simulink model "EngineModel_scaled_10_6_2016_dynamics"  (R2013a)
settings: Solver=ode4  StartTime=0.0  StopTime=30  FixedStep=0.2  RelTol=1e-3
values from neighbouring files (symbols this model uses):
  Fanmap_2 = [1 1 1 1 1 1 1 1 1 1 275.724 325.4224 ... (330 elements, 10x3x11)]    [enginemaps2.mat]
  HPCompmap_2 = [1 1 1 1 1 1 1 1 1 1 32.390865 37.6623195 ... (330 elements, 10x3x11)]    [enginemaps2.mat]
  HPTurbinemap_2 = [0.24979968 0.24979968 0.24979968 0.24979968 0.24979968 0.24979968 0.24979968 0.24979968 0.24979968 0.24979968 0.004250667 0.005047667 ... (330 elements, 10x3x11)]    [enginemaps2.mat]
  LPCompmap_2 = [1 1 1 1 1 1 1 1 1 1 34.17260994 40.23277722 ... (330 elements, 10x3x11)]    [enginemaps2.mat]
  LPTurbinemap_2 = [0.665969797 0.665969797 0.665969797 0.665969797 0.665969797 0.665969797 0.665969797 0.665969797 0.00912 0.013173333 0.015706667 0.01672 ... (264 elements, 8x3x11)]    [enginemaps2.mat]
undefined symbols (not defined in the file or in its folder): acc_or_dec, acceleration, Adiabatic_compression_fan, Adiabatic_compression_HPC, Adiabatic_compression_LPC, coldnozzle, compression_ram, cond_f2, D, datatables, deceleration, hotnozzle, HPT1, if_Nth, if_Ntl, if_Z, LPT, performancedynOL, thermo_combustor, transient, turbo
libraries: dspmtrx3 x8, aerolibatmos2 x6, dspsigattribs x3, dspsolvers x2, dspfactors x1
(part 1 of 10)
settings Model: Creator=BES  LastModifiedBy=BES
settings SolverCC: ZeroCrossAlgorithm=Adaptive
settings DataIOCC: InitialState=load('enginemaps1.mat')  LimitDataPoints=off

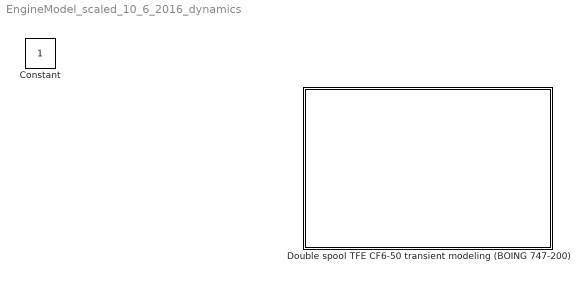
== system EngineModel_scaled_10_6_2016_dynamics ==
  Double spool TFE CF6-50 transient modeling (BOING 747-200) : Subsystem
      mask Display: image('b747.jpg')
  Constant : Constant  IOType=siggen

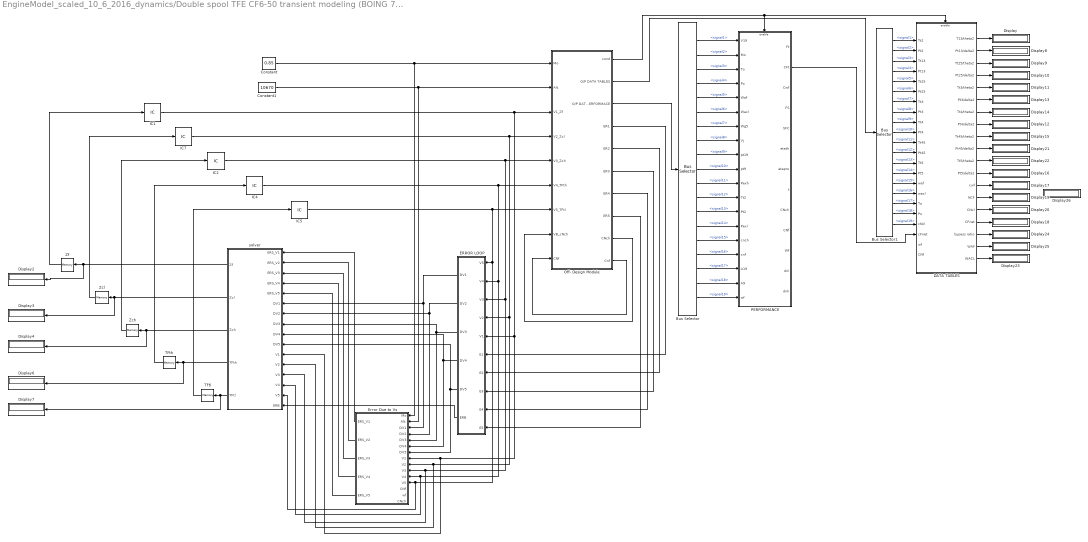
== system EngineModel_scaled_10_6_2016_dynamics/Double spool TFE CF6-50 transient modeling (BOING 747-200) ==
  Bus Selector : BusSelector  OutputSignals=signal1,signal2,signal3,signal4,signal5,signal6,signal7,signal8,signal9,signal10,signal11,signal12,signal13,signal14,signal15,signal16,signal17,signal18,signal19
  Bus Selector1 : BusSelector  OutputSignals=signal1,signal2,signal3,signal4,signal5,signal6,signal7,signal8,signal9,signal10,signal11,signal12,signal13,signal14,signal15,signal16,signal17,signal18,signal19
  Constant : Constant  Value=0.85
  Constant1 : Constant  Value=10670
  DATA TABLES : Subsystem
  Display{,2..4,6..26} (25 alike) : Display
  "ERROR LOOP " : Subsystem
  Error Due to Vs : Subsystem
  IC1 : InitialCondition  Value=0.838043
  IC2 : InitialCondition  Value=0.82992106
  IC4 : InitialCondition  Value=156.358278
  IC5 : InitialCondition  Value=677.9237033
  IC7 : InitialCondition  Value=0.8685268
  Off- Design Module : Subsystem
  PERFORMANCE : Subsystem
  TFth : Memory  X0=156
  TFtl : Memory  X0=674
  Zch : Memory  X0=0.83333
  Zcl : Memory  X0=0.83333
  Zf : Memory  X0=0.83333
  solver : Subsystem
  wires:
  Constant/1 -> Error Due to Vs/1(Mo), Off- Design Module/1(Mo)
  Constant1/1 -> Error Due to Vs/2(Alt.), Off- Design Module/2(Alt.)
  solver/1(Zf) -> Display2/1, Zf/1
  solver/2(Zcl) -> Display3/1, Zcl/1
  solver/3(Zch) -> Display4/1, Zch/1
  solver/4(TFth) -> TFth/1, Display6/1
  solver/5(TFtl) -> TFtl/1, Display7/1
  Off- Design Module/4(ER1) -> "ERROR LOOP "/6(E1)
  Off- Design Module/5(ER2) -> "ERROR LOOP "/7(E2)
  "ERROR LOOP "/6(ERB) -> solver/16(ERB)
  IC1/1 -> solver/11(V1), Error Due to Vs/8(V1), "ERROR LOOP "/5(V1), Off- Design Module/3(V1_Zf)
  IC7/1 -> solver/12(V2), Error Due to Vs/9(V2), "ERROR LOOP "/4(V2), Off- Design Module/4(V2_Zcl)
  IC2/1 -> solver/13(V3), Error Due to Vs/10(V3), "ERROR LOOP "/3(V3), Off- Design Module/5(V3_Zch)
  IC4/1 -> solver/14(V4), Error Due to Vs/11(V4), "ERROR LOOP "/2(V4), Off- Design Module/6(V4_TFth)
  IC5/1 -> solver/15(V5), Error Due to Vs/12(V5), "ERROR LOOP "/1(V5), Off- Design Module/7(V5_TFtl)
  Off- Design Module/1(cond) -> PERFORMANCE/Enable, DATA TABLES/Enable
  TFtl/1 -> IC5/1
  TFth/1 -> IC4/1
  Zch/1 -> IC2/1
  Zcl/1 -> IC7/1
  Zf/1 -> IC1/1
  Off- Design Module/2(O/P DATA TABLES) -> Bus Selector1/1
  Bus Selector1/1 -> DATA TABLES/1(Tt2)  "<signal1>"
  Bus Selector1/2 -> DATA TABLES/2(Pt2)  "<signal2>"
  Bus Selector1/3 -> DATA TABLES/3(Tt13)  "<signal3>"
  Bus Selector1/4 -> DATA TABLES/4(Pt13)  "<signal4>"
  Bus Selector1/5 -> DATA TABLES/5(Tt25)  "<signal5>"
  Bus Selector1/6 -> DATA TABLES/6(Pt25)  "<signal6>"
  Bus Selector1/7 -> DATA TABLES/7(Tt3)  "<signal7>"
  Bus Selector1/8 -> DATA TABLES/8(Pt3)  "<signal8>"
  Bus Selector1/9 -> DATA TABLES/9(Tt4)  "<signal9>"
  Bus Selector1/10 -> DATA TABLES/10(Pt4)  "<signal10>"
  Bus Selector1/11 -> DATA TABLES/11(Tt45)  "<signal11>"
  Bus Selector1/12 -> DATA TABLES/12(Pt45)  "<signal12>"
  Bus Selector1/13 -> DATA TABLES/13(Tt5)  "<signal13>"
  Bus Selector1/14 -> DATA TABLES/14(Pt5)  "<signal14>"
  Bus Selector1/15 -> DATA TABLES/15(waf)  "<signal15>"
  Bus Selector1/16 -> DATA TABLES/16(wacl)  "<signal16>"
  Bus Selector1/17 -> DATA TABLES/17(To)  "<signal17>"
  Bus Selector1/18 -> DATA TABLES/18(Po)  "<signal18>"
  Bus Selector1/19 -> DATA TABLES/19(cNcl)  "<signal19>"
  PERFORMANCE/2(CFt) -> DATA TABLES/20(cFnet)
  DATA TABLES/1(T13/theta2) -> Display/1
  DATA TABLES/2(Pt13/delta2) -> Display8/1
  DATA TABLES/3(Tt25/theta2) -> Display9/1
  DATA TABLES/4(Pt25/delta2) -> Display10/1
  DATA TABLES/5(Tt3/theta2) -> Display11/1
  DATA TABLES/6(Pt3/delta2) -> Display13/1
  DATA TABLES/7(Tt4/theta2) -> Display14/1
  DATA TABLES/8(Pt4/delta2) -> Display12/1
  DATA TABLES/9(Tt45/theta2) -> Display15/1
  DATA TABLES/10(Pt45/delta2) -> Display21/1
  DATA TABLES/11(Tt5/theta2) -> Display22/1
  DATA TABLES/12(Pt5/delta2) -> Display16/1
  DATA TABLES/13(cwf) -> Display17/1
  DATA TABLES/14(NCF) -> Display19/1
  DATA TABLES/15(CNcl) -> Display20/1
  DATA TABLES/16(CFnet) -> Display18/1
  DATA TABLES/17(bypass ratio) -> Display24/1
  DATA TABLES/18(WAF) -> Display25/1
  DATA TABLES/19(WACL) -> Display23/1
  Off- Design Module/6(ER3) -> "ERROR LOOP "/8(E3)
  Off- Design Module/7(ER4) -> "ERROR LOOP "/9(E4)
  Off- Design Module/8(ER5) -> "ERROR LOOP "/10(E5)
  "ERROR LOOP "/1(DV1) -> solver/6(DV1), Error Due to Vs/3(DV1)
  "ERROR LOOP "/2(DV2) -> solver/7(DV2), Error Due to Vs/4(DV2)
  "ERROR LOOP "/5(DV5) -> solver/10(DV5), Error Due to Vs/7(DV5)
  "ERROR LOOP "/4(DV4) -> solver/9(DV4), Error Due to Vs/6(DV4)
  "ERROR LOOP "/3(DV3) -> solver/8(DV3), Error Due to Vs/5(DV3)
  Error Due to Vs/1(ERS_V1) -> solver/1(ERS_V1)
  Error Due to Vs/2(ERS_V2) -> solver/2(ERS_V2)
  Error Due to Vs/3(ERS_V3) -> solver/3(ERS_V3)
  Error Due to Vs/4(ERS_V4) -> solver/4(ERS_V4)
  Error Due to Vs/5(ERS_V5) -> solver/5(ERS_V5)
  Bus Selector/1 -> PERFORMANCE/1(V19)  "<signal1>"
  Bus Selector/2 -> PERFORMANCE/2(Mo)  "<signal2>"
  Bus Selector/3 -> PERFORMANCE/3(To)  "<signal3>"
  Bus Selector/4 -> PERFORMANCE/4(Po)  "<signal4>"
  Bus Selector/5 -> PERFORMANCE/5(Waf)  "<signal5>"
  Bus Selector/6 -> PERFORMANCE/6(Wacl)  "<signal6>"
  Bus Selector/7 -> PERFORMANCE/7(Wg5)  "<signal7>"
  Bus Selector/8 -> PERFORMANCE/8(Vj)  "<signal8>"
  Bus Selector/9 -> PERFORMANCE/9(pt19)  "<signal9>"
  Bus Selector/10 -> PERFORMANCE/10(pt9)  "<signal10>"
  Bus Selector/11 -> PERFORMANCE/11(Pexh)  "<signal11>"
  Bus Selector/12 -> PERFORMANCE/12(Tt2)  "<signal12>"
  Bus Selector/13 -> PERFORMANCE/13(Pt2)  "<signal13>"
  Bus Selector/14 -> PERFORMANCE/14(Pexl)  "<signal14>"
  Bus Selector/15 -> PERFORMANCE/15(cnch)  "<signal15>"
  Bus Selector/16 -> PERFORMANCE/16(cnf)  "<signal16>"
  Bus Selector/17 -> PERFORMANCE/17(A19)  "<signal17>"
  Bus Selector/18 -> PERFORMANCE/18(A9)  "<signal18>"
  Bus Selector/19 -> PERFORMANCE/19(wf)  "<signal19>"
  Off- Design Module/3(O/P DATA FOR PERFORMACE) -> Bus Selector/1
  Off- Design Module/10(Cnf) -> Off- Design Module/9(CNf)
  Off- Design Module/9(CNch) -> Off- Design Module/8(VB_cNch)

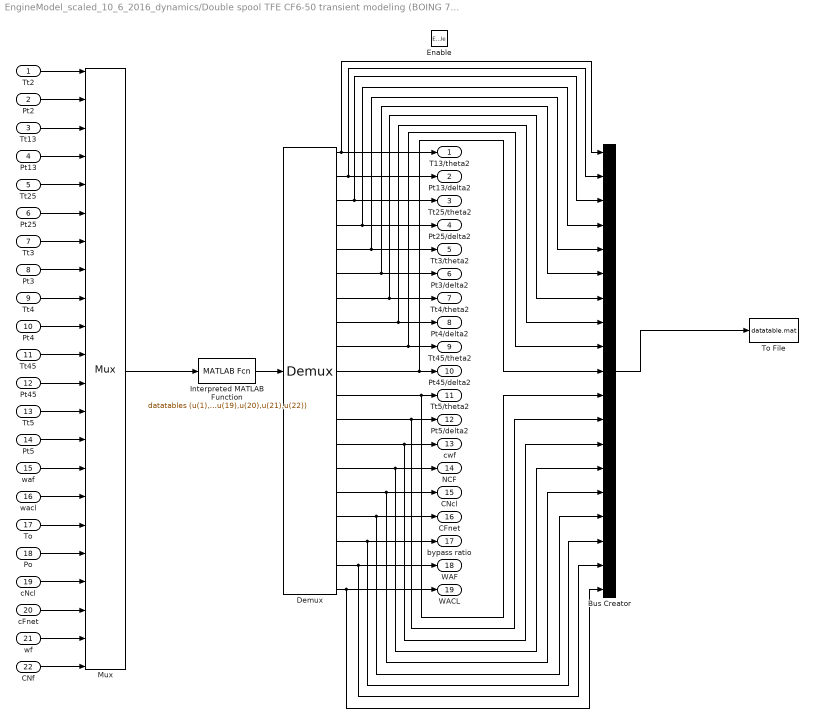
== system EngineModel_scaled_10_6_2016_dynamics/Double spool TFE CF6-50 transient modeling (BOING 747-200)/DATA TABLES ==
  Tt2 : Inport
  Pt2 : Inport  Port=2
  Tt13 : Inport  Port=3
  Pt13 : Inport  Port=4
  Tt25 : Inport  Port=5
  Pt25 : Inport  Port=6
  Tt3 : Inport  Port=7
  Pt3 : Inport  Port=8
  Tt4 : Inport  Port=9
  Pt4 : Inport  Port=10
  Tt45 : Inport  Port=11
  Pt45 : Inport  Port=12
  Tt5 : Inport  Port=13
  Pt5 : Inport  Port=14
  waf : Inport  Port=15
  wacl : Inport  Port=16
  To : Inport  Port=17
  Po : Inport  Port=18
  cNcl : Inport  Port=19
  cFnet : Inport  Port=20
  wf : Inport  Port=21
  CNf : Inport  Port=22
  Enable : EnablePort  StatesWhenEnabling=reset
  Bus Creator : BusCreator  Inputs=19
  Demux : Demux  Outputs=19
  Interpreted MATLAB Function : MATLABFcn  MATLABFcn=datatables (u(1),u(2),u(3),u(4),u(5),u(6),u(7),u(8),u(9),u(10),u(11),u(12),u(13),u(14),u(15),u(16),u(17),u(18),u(19),u(20),u(21),u(22))  OutputDimensions=19
  Mux : Mux  Inputs=22
      settings: DisplayOption=signals
  To File : ToFile  Filename=datatable.mat  MatrixName=bes
  T13/theta2 : Outport
  Pt13/delta2 : Outport  Port=2
  Tt25/theta2 : Outport  Port=3
  Pt25/delta2 : Outport  Port=4
  Tt3/theta2 : Outport  Port=5
  Pt3/delta2 : Outport  Port=6
  Tt4/theta2 : Outport  Port=7
  Pt4/delta2 : Outport  Port=8
  Tt45/theta2 : Outport  Port=9
  Pt45/delta2 : Outport  Port=10
  Tt5/theta2 : Outport  Port=11
  Pt5/delta2 : Outport  Port=12
  cwf : Outport  Port=13
  NCF : Outport  Port=14
  CNcl : Outport  Port=15
  CFnet : Outport  Port=16
  bypass ratio : Outport  Port=17
  WAF : Outport  Port=18
  WACL : Outport  Port=19
  wires:
  Pt5/1 -> Mux/14
  Tt5/1 -> Mux/13
  Pt45/1 -> Mux/12
  Tt45/1 -> Mux/11
  Pt4/1 -> Mux/10
  Pt3/1 -> Mux/8
  Tt3/1 -> Mux/7
  Pt25/1 -> Mux/6
  Tt25/1 -> Mux/5
  Pt13/1 -> Mux/4
  Tt13/1 -> Mux/3
  Pt2/1 -> Mux/2
  Tt2/1 -> Mux/1
  Interpreted MATLAB Function/1 -> Demux/1
  Mux/1 -> Interpreted MATLAB Function/1
  waf/1 -> Mux/15
  cNcl/1 -> Mux/19
  wacl/1 -> Mux/16
  To/1 -> Mux/17
  Po/1 -> Mux/18
  cFnet/1 -> Mux/20
  wf/1 -> Mux/21
  CNf/1 -> Mux/22
  Demux/1 -> Bus Creator/1, T13/theta2/1
  Demux/4 -> Bus Creator/4, Pt25/delta2/1
  Demux/5 -> Bus Creator/5, Tt3/theta2/1
  Demux/6 -> Bus Creator/6, Pt3/delta2/1
  Demux/7 -> Bus Creator/7, Tt4/theta2/1
  Demux/8 -> Bus Creator/8, Pt4/delta2/1
  Demux/9 -> Bus Creator/9, Tt45/theta2/1
  Demux/11 -> Bus Creator/11, Tt5/theta2/1
  Demux/12 -> Bus Creator/12, Pt5/delta2/1
  Demux/13 -> Bus Creator/13, cwf/1
  Demux/14 -> Bus Creator/14, NCF/1
  Demux/15 -> Bus Creator/15, CNcl/1
  Demux/16 -> Bus Creator/16, CFnet/1
  Demux/17 -> Bus Creator/17, bypass ratio/1
  Demux/18 -> Bus Creator/18, WAF/1
  Demux/19 -> Bus Creator/19, WACL/1
  Demux/2 -> Bus Creator/2, Pt13/delta2/1
  Bus Creator/1 -> To File/1
  Demux/3 -> Bus Creator/3, Tt25/theta2/1
  Demux/10 -> Bus Creator/10, Pt45/delta2/1
  Tt4/1 -> Mux/9

== system EngineModel_scaled_10_6_2016_dynamics/Double spool TFE CF6-50 transient modeling (BOING 747-200)/ERROR LOOP  ==
  V5 : Inport
  V4 : Inport  Port=2
  V3 : Inport  Port=3
  V2 : Inport  Port=4
  V1 : Inport  Port=5
  E1 : Inport  Port=6
  E2 : Inport  Port=7
  E3 : Inport  Port=8
  E4 : Inport  Port=9
  E5 : Inport  Port=10
  Constant : Constant  Value=0.005
  Constant1 : Constant  Value=100
  Display1 : Display
  Divide : Product  Inputs=*/
  Divide1 : Product  Inputs=*/
  Product{,1,3..5} (5 alike) : Product
  Vector Concatenate : Concatenate  NumInputs=5  Mode=Multidimensional array
  DV1 : Outport
  DV2 : Outport  Port=2
  DV3 : Outport  Port=3
  DV4 : Outport  Port=4
  DV5 : Outport  Port=5
  ERB : Outport  Port=6
  wires:
  Constant/1 -> Product5/1, Product4/1, Product3/1, Product1/1, Product/1
  V1/1 -> Product5/2
  V2/1 -> Product4/2
  V3/1 -> Product3/2
  Product3/1 -> DV3/1
  Product4/1 -> DV2/1
  Product5/1 -> DV1/1
  E1/1 -> Vector Concatenate/1
  E2/1 -> Vector Concatenate/2
  E3/1 -> Vector Concatenate/3
  E4/1 -> Vector Concatenate/4
  E5/1 -> Vector Concatenate/5
  Vector Concatenate/1 -> ERB/1, Display1/1
  Product/1 -> DV5/1
  Product1/1 -> DV4/1
  V5/1 -> Divide/1
  Constant1/1 -> Divide1/2, Divide/2
  Divide/1 -> Product/2
  V4/1 -> Divide1/1
  Divide1/1 -> Product1/2

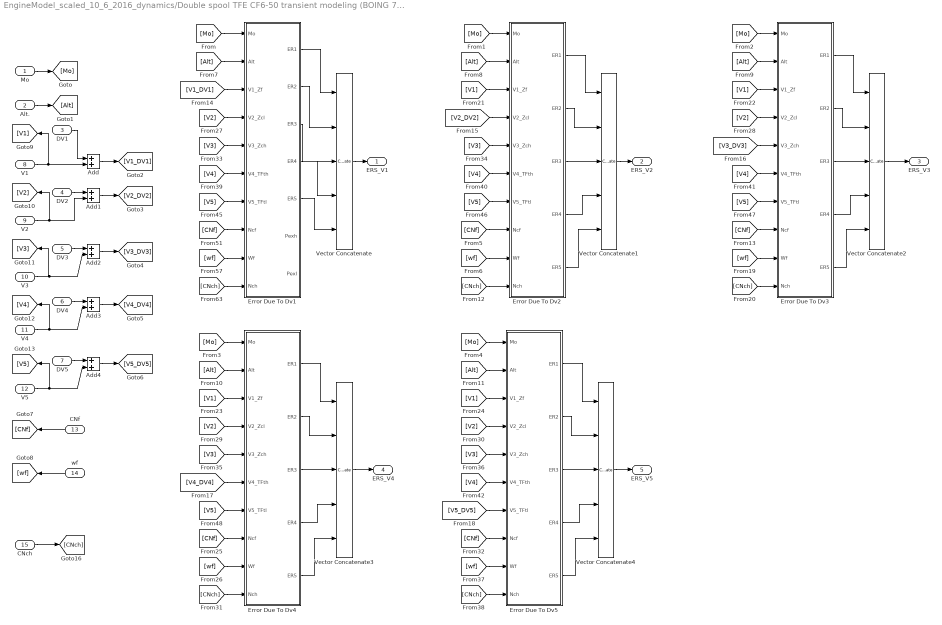
== system EngineModel_scaled_10_6_2016_dynamics/Double spool TFE CF6-50 transient modeling (BOING 747-200)/Error Due to Vs ==
  Mo : Inport
  Alt. : Inport  Port=2
  DV1 : Inport  Port=3
  DV2 : Inport  Port=4
  DV3 : Inport  Port=5
  DV4 : Inport  Port=6
  DV5 : Inport  Port=7
  V1 : Inport  Port=8
  V2 : Inport  Port=9
  V3 : Inport  Port=10
  V4 : Inport  Port=11
  V5 : Inport  Port=12
  CNf : Inport  Port=13
  wf : Inport  Port=14
  CNch : Inport  Port=15
  Add{,1..4} (5 alike) : Sum
  Error Due To Dv1 : Subsystem
  Error Due To Dv2 : Subsystem
  Error Due To Dv3 : Subsystem
  Error Due To Dv4 : Subsystem
  Error Due To Dv5 : Subsystem
  Vector Concatenate{,1..4} (5 alike) : Concatenate  NumInputs=5
  ERS_V1 : Outport
  ERS_V2 : Outport  Port=2
  ERS_V3 : Outport  Port=3
  ERS_V4 : Outport  Port=4
  ERS_V5 : Outport  Port=5
  wires:
  Vector Concatenate/1 -> ERS_V1/1
  Error Due To Dv1/1(ER1) -> Vector Concatenate/1
  Error Due To Dv1/2(ER2) -> Vector Concatenate/2
  Error Due To Dv1/4(ER4) -> Vector Concatenate/4
  Error Due To Dv1/5(ER5) -> Vector Concatenate/5
  DV1/1 -> Add/1
  V1/1 -> [V1], Add/2
  DV2/1 -> Add1/1
  DV3/1 -> Add2/1
  DV4/1 -> Add3/1
  DV5/1 -> Add4/1
  Mo/1 -> [Mo]
  [Mo] -> Error Due To Dv1/1(Mo)
  [Mo] -> Error Due To Dv2/1(Mo)
  [Mo] -> Error Due To Dv3/1(Mo)
  [Mo] -> Error Due To Dv4/1(Mo)
  [Mo] -> Error Due To Dv5/1(Mo)
  [Alt] -> Error Due To Dv1/2(Alt)
  Alt./1 -> [Alt]
  [Alt] -> Error Due To Dv2/2(Alt)
  [Alt] -> Error Due To Dv3/2(Alt)
  [Alt] -> Error Due To Dv4/2(Alt)
  [Alt] -> Error Due To Dv5/2(Alt)
  Add/1 -> [V1_DV1]
  Add1/1 -> [V2_DV2]
  Add2/1 -> [V3_DV3]
  Add3/1 -> [V4_DV4]
  Add4/1 -> [V5_DV5]
  [V2_DV2] -> Error Due To Dv2/4(V2_Zcl)
  [V3_DV3] -> Error Due To Dv3/5(V3_Zch)
  [V4_DV4] -> Error Due To Dv4/6(V4_TFth)
  [V5_DV5] -> Error Due To Dv5/7(V5_TFtl)
  V2/1 -> [V2], Add1/2
  V3/1 -> [V3], Add2/2
  V4/1 -> [V4], Add3/2
  V5/1 -> [V5], Add4/2
  CNch/1 -> [CNch]
  [V1] -> Error Due To Dv2/3(V1_Zf)
  [V1] -> Error Due To Dv3/3(V1_Zf)
  [V1] -> Error Due To Dv4/3(V1_Zf)
  [V1] -> Error Due To Dv5/3(V1_Zf)
  [V2] -> Error Due To Dv3/4(V2_Zcl)
  [V2] -> Error Due To Dv4/4(V2_Zcl)
  [V2] -> Error Due To Dv5/4(V2_Zcl)
  [V3] -> Error Due To Dv2/5(V3_Zch)
  [V3] -> Error Due To Dv4/5(V3_Zch)
  [V3] -> Error Due To Dv5/5(V3_Zch)
  [V4] -> Error Due To Dv2/6(V4_TFth)
  [V4] -> Error Due To Dv3/6(V4_TFth)
  [V4] -> Error Due To Dv5/6(V4_TFth)
  [V5] -> Error Due To Dv2/7(V5_TFtl)
  [V5] -> Error Due To Dv3/7(V5_TFtl)
  [V5] -> Error Due To Dv4/7(V5_TFtl)
  [CNf] -> Error Due To Dv2/8(Ncf)
  [CNf] -> Error Due To Dv3/8(Ncf)
  [CNf] -> Error Due To Dv4/8(Ncf)
  [CNf] -> Error Due To Dv5/8(Ncf)
  [wf] -> Error Due To Dv2/9(Wf)
  [wf] -> Error Due To Dv3/9(Wf)
  [wf] -> Error Due To Dv4/9(Wf)
  [wf] -> Error Due To Dv5/9(Wf)
  [CNch] -> Error Due To Dv2/10(Nch)
  [CNch] -> Error Due To Dv3/10(Nch)
  [CNch] -> Error Due To Dv4/10(Nch)
  [CNch] -> Error Due To Dv5/10(Nch)
  [V1_DV1] -> Error Due To Dv1/3(V1_Zf)
  [V2] -> Error Due To Dv1/4(V2_Zcl)
  [V3] -> Error Due To Dv1/5(V3_Zch)
  [V4] -> Error Due To Dv1/6(V4_TFth)
  [V5] -> Error Due To Dv1/7(V5_TFtl)
  [CNf] -> Error Due To Dv1/8(Ncf)
  [wf] -> Error Due To Dv1/9(Wf)
  [CNch] -> Error Due To Dv1/10(Nch)
  Error Due To Dv1/3(ER3) -> Vector Concatenate/3
  Vector Concatenate1/1 -> ERS_V2/1
  Error Due To Dv2/1(ER1) -> Vector Concatenate1/1
  Error Due To Dv2/2(ER2) -> Vector Concatenate1/2
  Error Due To Dv2/4(ER4) -> Vector Concatenate1/4
  Error Due To Dv2/5(ER5) -> Vector Concatenate1/5
  Error Due To Dv2/3(ER3) -> Vector Concatenate1/3
  Error Due To Dv3/1(ER1) -> Vector Concatenate2/1
  Error Due To Dv3/2(ER2) -> Vector Concatenate2/2
  Error Due To Dv3/4(ER4) -> Vector Concatenate2/4
  Error Due To Dv3/5(ER5) -> Vector Concatenate2/5
  Error Due To Dv3/3(ER3) -> Vector Concatenate2/3
  Vector Concatenate2/1 -> ERS_V3/1
  Error Due To Dv4/1(ER1) -> Vector Concatenate3/1
  Error Due To Dv4/2(ER2) -> Vector Concatenate3/2
  Error Due To Dv4/4(ER4) -> Vector Concatenate3/4
  Error Due To Dv4/5(ER5) -> Vector Concatenate3/5
  Error Due To Dv4/3(ER3) -> Vector Concatenate3/3
  Vector Concatenate3/1 -> ERS_V4/1
  Error Due To Dv5/1(ER1) -> Vector Concatenate4/1
  Error Due To Dv5/2(ER2) -> Vector Concatenate4/2
  Error Due To Dv5/4(ER4) -> Vector Concatenate4/4
  Error Due To Dv5/5(ER5) -> Vector Concatenate4/5
  Error Due To Dv5/3(ER3) -> Vector Concatenate4/3
  Vector Concatenate4/1 -> ERS_V5/1
  CNf/1 -> [CNf]
  wf/1 -> [wf]

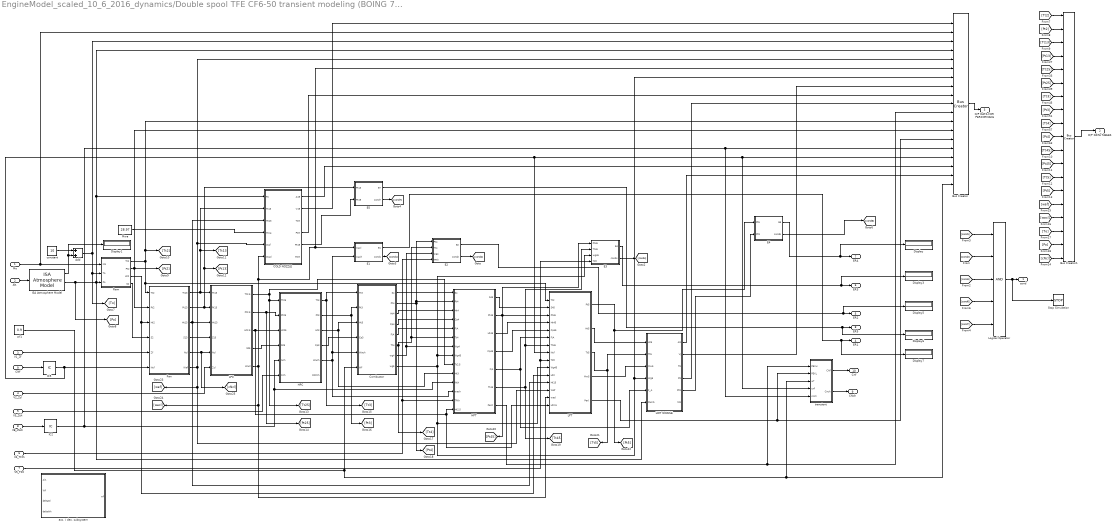
== system EngineModel_scaled_10_6_2016_dynamics/Double spool TFE CF6-50 transient modeling (BOING 747-200)/Off- Design Module ==
  Mo : Inport
  Alt. : Inport  Port=2
  V1_Zf : Inport  Port=3
  V2_Zcl : Inport  Port=4
  V3_Zch : Inport  Port=5
  V4_TFth : Inport  Port=6
  V5_TFtl : Inport  Port=7
  VB_cNch : Inport  Port=8
  CNf : Inport  Port=9
  Add : Sum
  Bus Creator : BusCreator  Inputs=19
  Bus Creator1 : BusCreator  Inputs=19
  COLD NOZZLE : Subsystem
  Combustor : Subsystem
  Display{,1,3,5..7} (6 alike) : Display
  E1 : Subsystem
  E2 : Subsystem
  E3 : Subsystem
  E4 : Subsystem
  E5 : Subsystem
  Fan : Subsystem
  HOT NOZZLE : Subsystem
  HPC : Subsystem
  HPT : Subsystem
  IC2 : InitialCondition
  IC5 : InitialCondition  Value=1.0141259
  ISA Atmosphere Model : aerolibatmos2/ISA Atmosphere Model  custom=on  g=9.8  gamma=1.4  R=287.0531  L=0.0065  h_trop=11000  h_strat=20000  rho0=1.225  P0=101325  T0=288.15  h0=0
  LPC : Subsystem
  LPT : Subsystem
  Logical Operator : Logic  Inputs=5  IconShape=distinctive  AllPortsSameDT=off  OutDataTypeStr=boolean
  Mwa : Constant  Value=28.97
  Ram : Subsystem
  Stop Simulation : Stop
  acc. / dec. subsystem : Subsystem
  constant : Constant  Value=10
  transient : Subsystem
  wf1 : Constant  Value=0.9
  cond : Outport
  O/P DATA TABLES : Outport  Port=2
  O/P DATA FOR PERFORMACE : Outport  Port=3
  ER1 : Outport  Port=4
  ER2 : Outport  Port=5
  ER3 : Outport  Port=6
  ER4 : Outport  Port=7
  ER5 : Outport  Port=8
  CNch : Outport  Port=9
  Cnf : Outport  Port=10
  wires:
  Alt./1 -> ISA Atmosphere Model/1
  Mo/1 -> Bus Creator/2, Ram/1(Mo)
  Add/1 -> Bus Creator/3, [To], Ram/2(To)
  ISA Atmosphere Model/3 -> [Po], HOT NOZZLE/6(Pamb), Ram/3(Po), Bus Creator/4, COLD NOZZLE/1(Po)
  constant/1 -> Add/1
  Ram/1(Tt2) -> [Tt2], Bus Creator/12, Fan/1(Tt2), LPT/1(Tt2)
  Ram/2(Pt2) -> [Pt2], Bus Creator/13, Fan/2(Pt2)
  HPC/2(Pt3) -> [Pt3], Combustor/2(Pt3)
  HPC/3(Ht3) -> HPT/10(Ht3), Combustor/3(Ht3)
  Combustor/2(Pt4) -> [Pt4], E2/1(Pt4), HPT/2(Pt4)
  Combustor/4(Cp4) -> HPT/4(Cp4)
  Combustor/5(F/A) -> HPT/5(F/A)
  Combustor/6(Tt4) -> [Tt4], E2/2(Tt4), HPT/6(Tt4)
  LPT/2(Ht5) -> HOT NOZZLE/1(Ht5)
  LPT/3(Tt5) -> [Tt5], HOT NOZZLE/2(Tt5)
  V1_Zf/1 -> Fan/5(Zf)
  V2_Zcl/1 -> LPC/6(Zcl)
  V3_Zch/1 -> HPC/6(Zch)
  VB_cNch/1 -> IC2/1
  V4_TFth/1 -> E2/4(TFth), HPT/13(TFth)
  Combustor/7(wg4) -> E2/3(wg4), HPT/7(Wg4)
  LPT/4(Mw5) -> HOT NOZZLE/3(Mw5)
  Fan/3(Ht13) -> LPC/3(Ht13), LPT/12(Ht13), COLD NOZZLE/3(Ht13)
  Mwa/1 -> COLD NOZZLE/4(Mwa)
  Fan/6(Waf) -> LPT/13(Waf), [waf], Bus Creator/5, COLD NOZZLE/5(Waf)
  LPC/5(Wacl) -> COLD NOZZLE/6(Wacl), Bus Creator/6, E1/1(wacl), LPT/14(wacl), [wacl]
  COLD NOZZLE/5(Pt19) -> E5/2(Pt19)
  LPC/3(Ht2.5) -> LPT/15(Ht2.5), HPT/14(Ht2.5), HPC/3(Ht25)
  LPT/1(Pt5) -> [Pt5], E4/1(Pt5)
  HOT NOZZLE/5(Pt9) -> E4/2(Pt9)
  Combustor/8(wg5) -> LPT/10(Wg45), Bus Creator/7, HOT NOZZLE/4(Wg5), E3/3(wg45), HPT/8(Wg45)
  Combustor/3(Ht4) -> HPT/3(Ht4)
  Combustor/1(S4) -> HPT/1(S4)
  Ram/4(S2) -> Fan/4(S2)
  Fan/5(Ncl) -> [cNcl], LPC/5(Ncl)
  Fan/4(S13) -> LPC/4(S13)
  LPC/4(S25) -> HPC/4(S25)
  HPC/5(Wach) -> HPT/12(wach), E1/2(wach), Combustor/5(Wach)
  HPT/1(S45) -> LPT/2(S45)
  HPT/2(Pt45) -> [Pt45], LPT/3(Pt45), E3/1(Pt45)
  HPT/3(Ht45) -> LPT/4(Ht45)
  HPT/4(Cp45) -> LPT/5(Cp45)
  HPT/6(Tt45) -> [Tt45], E3/2(Tt45), LPT/7(Tt45)
  V5_TFtl/1 -> E3/4(TFtl), LPT/9(TFtl)
  E4/1(E6) -> Display/1, ER4/1
  E3/1(E4) -> Display3/1, ER3/1
  E2/1(E2) -> Display5/1, ER2/1
  E5/1(E7) -> Display6/1, ER5/1
  E1/1(E1) -> Display7/1, ER1/1
  HOT NOZZLE/2(Vj) -> Bus Creator/8
  COLD NOZZLE/4(P19) -> Bus Creator/9
  HOT NOZZLE/4(P9) -> Bus Creator/10
  ISA Atmosphere Model/1 -> Display1/1, Add/2
  HOT NOZZLE/1(A9) -> Bus Creator/18
  COLD NOZZLE/2(V19) -> Bus Creator/1
  Bus Creator/1 -> O/P DATA FOR PERFORMACE/1
  E4/2(cond6) -> [cond6]
  E3/2(cond4) -> [cond4]
  E2/2(cond2) -> [cond2]
  E1/2(cond1) -> [cond1]
  E5/2("cond7 ") -> [cond7]
  Logical Operator/1 -> Stop Simulation/1, cond/1
  HPC/4(Cp3) -> Combustor/4(Cp3)
  [Tt2] -> Bus Creator1/1
  [Pt2] -> Bus Creator1/2
  [Tt13] -> Bus Creator1/3
  [Pt13] -> Bus Creator1/4
  [Tt25] -> Bus Creator1/5
  [Pt25] -> Bus Creator1/6
  [Tt3] -> Bus Creator1/7
  [Pt3] -> Bus Creator1/8
  [Tt4] -> Bus Creator1/9
  [Pt4] -> Bus Creator1/10
  [Tt45] -> Bus Creator1/11
  [Pt45] -> Bus Creator1/12
  [Tt5] -> Bus Creator1/13
  [Pt5] -> Bus Creator1/14
  [waf] -> Bus Creator1/15
  [wacl] -> Bus Creator1/16
  [To] -> Bus Creator1/17
  [Po] -> Bus Creator1/18
  Fan/1(Tt13) -> LPC/1(Tt13), [Tt13], COLD NOZZLE/2(Tt13)
  Fan/2(Pt13) -> [Pt13], E5/1(Pt13), LPC/2(Pt13)
  LPC/1(Tt2.5) -> HPT/9(Tt2.5), [Tt25], HPC/1(Tt25)
  LPC/2(Pt2.5) -> [Pt25], HPC/2(Pt25)
  HPC/1(Tt3) -> [Tt3], Combustor/1(Tt3)
  Bus Creator1/1 -> O/P DATA TABLES/1
  [cNcl] -> Bus Creator1/19
  HPT/5(F\A) -> HOT NOZZLE/5(F_A), LPT/6(F/A)
  [cond2] -> Logical Operator/2
  [cond1] -> Logical Operator/1
  [cond4] -> Logical Operator/3
  [cond6] -> Logical Operator/4
  [cond7] -> Logical Operator/5
  Ram/3(Ht2) -> Fan/3(Ht2), LPT/11(Ht2)
  CNf/1 -> IC5/1
  IC2/1 -> transient/5(cnch), Bus Creator/15, HPC/5(Nch), HPT/11(Nch)
  LPT/5(Pexl) -> transient/2(PEXL), Bus Creator/14
  wf1/1 -> transient/3(wf), Bus Creator/19, Combustor/6(Wf)
  COLD NOZZLE/1(A19) -> Bus Creator/17
  HPT/7(Pexh) -> transient/1(PEXH), Bus Creator/11
  IC5/1 -> LPT/8(Ncf), transient/4(cnf), Bus Creator/16, Fan/6(Ncf)
  transient/1(CNf) -> Cnf/1
  transient/2(Cnch) -> CNch/1

== system EngineModel_scaled_10_6_2016_dynamics/Double spool TFE CF6-50 transient modeling (BOING 747-200)/PERFORMANCE ==
  V19 : Inport
  Mo : Inport  Port=2
  To : Inport  Port=3
  Po : Inport  Port=4
  Waf : Inport  Port=5
  Wacl : Inport  Port=6
  Wg5 : Inport  Port=7
  Vj : Inport  Port=8
  pt19 : Inport  Port=9
  pt9 : Inport  Port=10
  Pexh : Inport  Port=11
  Tt2 : Inport  Port=12
  Pt2 : Inport  Port=13
  Pexl : Inport  Port=14
  cnch : Inport  Port=15
  cnf : Inport  Port=16
  A19 : Inport  Port=17
  A9 : Inport  Port=18
  wf : Inport  Port=19
  Enable : EnablePort  StatesWhenEnabling=reset
  Bus Creator : BusCreator  Inputs=6
  Demux : Demux  Outputs=13
  Interpreted MATLAB Function : MATLABFcn  MATLABFcn=performancedynOL(u(1),u(2),u(3),u(4),u(5),u(6),u(7),u(8),u(9),u(10),u(11),u(12),u(13),u(14),u(15),u(16),u(17),u(18),u(19),u(20),u(21),u(22))  OutputDimensions=13
  Mux : Mux  Inputs=22
      settings: DisplayOption=signals
  To File : ToFile  Filename=datatabledyn1.mat  MatrixName=bas1
  Ft : Outport
  CFt : Outport  Port=2
  Cwf : Outport  Port=3
  FS : Outport  Port=4
  SFC : Outport  Port=5
  etath : Outport  Port=6
  etapro : Outport  Port=7
  t : Outport  Port=8
  CNch : Outport  Port=9
  CNf : Outport  Port=10
  Wf : Outport  Port=11
  dnl : Outport  Port=12
  dnh : Outport  Port=13
  wires:
  Mux/1 -> Interpreted MATLAB Function/1
  Interpreted MATLAB Function/1 -> Demux/1
  V19/1 -> Mux/1
  Mo/1 -> Mux/2
  To/1 -> Mux/3
  Po/1 -> Mux/4
  Waf/1 -> Mux/5
  Wacl/1 -> Mux/6
  Wg5/1 -> Mux/7
  Vj/1 -> Mux/8
  pt19/1 -> Mux/9
  pt9/1 -> Mux/10
  Pexh/1 -> Mux/11
  Tt2/1 -> Mux/12
  Pt2/1 -> Mux/13
  Pexl/1 -> Mux/14
  cnch/1 -> Mux/15
  cnf/1 -> Mux/16
  A19/1 -> Mux/17
  A9/1 -> Mux/18
  wf/1 -> Mux/19
  Bus Creator/1 -> To File/1
  Demux/1 -> Ft/1
  Demux/2 -> CFt/1
  Demux/3 -> Cwf/1
  Demux/4 -> FS/1
  Demux/5 -> SFC/1
  Demux/6 -> etath/1
  Demux/7 -> etapro/1
  Demux/8 -> dnl/1
  Demux/9 -> dnh/1
  Demux/10 -> CNch/1
  Demux/11 -> CNf/1
  Demux/12 -> Wf/1
  Demux/13 -> t/1

== system EngineModel_scaled_10_6_2016_dynamics/Double spool TFE CF6-50 transient modeling (BOING 747-200)/solver ==
  ERS_V1 : Inport
  ERS_V2 : Inport  Port=2
  ERS_V3 : Inport  Port=3
  ERS_V4 : Inport  Port=4
  ERS_V5 : Inport  Port=5
  DV1 : Inport  Port=6
  DV2 : Inport  Port=7
  DV3 : Inport  Port=8
  DV4 : Inport  Port=9
  DV5 : Inport  Port=10
  V1 : Inport  Port=11
  V2 : Inport  Port=12
  V3 : Inport  Port=13
  V4 : Inport  Port=14
  V5 : Inport  Port=15
  ERB : Inport  Port=16
  " LU Inverse" : Subsystem  AncestorBlock=dspinverses/ LU Inverse  mask(LU Inverse){}
      mask help: Matrix inverse using LU factorization.
      mask Help: eval('blocksethelp');
      mask Display:
      | text(0.25,0.85,'General')
      | text(0.25,0.70,'Inverse')
      | text(0.35,0.25,'(LU)')
  Add{,1..4} (5 alike) : Sum
  Constant : Constant  Value=0.1
  Constant1 : Constant  Value=0
  Demux : Demux  Outputs=5
  Display{,1..2,4} (4 alike) : Display
  EMAT Concatenate : Concatenate  NumInputs=5  Mode=Multidimensional array  ConcatenateDimension=2
  EMAT New : Subsystem
  Matrix Multiply : Product  Multiplication=Matrix(*)
  Product : Product
  Subtract : Sum  Inputs=+-
  Zf : Outport
  Zcl : Outport  Port=2
  Zch : Outport  Port=3
  TFth : Outport  Port=4
  TFtl : Outport  Port=5
  wires:
  V1/1 -> Add/2
  V2/1 -> Add1/2
  V3/1 -> Add2/2
  V4/1 -> Add3/2
  V5/1 -> Add4/2
  " LU Inverse"/1(inv(A)) -> Matrix Multiply/1, Display1/1
  EMAT Concatenate/1 -> " LU Inverse"/1(A), Display/1
  Constant/1 -> Product/1
  Constant1/1 -> Subtract/1
  Matrix Multiply/1 -> Product/2, Display2/1
  Product/1 -> Demux/1, Display4/1
  Demux/1 -> Add/1
  Demux/2 -> Add1/1
  Demux/3 -> Add2/1
  Demux/4 -> Add3/1
  Demux/5 -> Add4/1
  ERS_V1/1 -> EMAT New/1(ERS_V1)
  ERS_V2/1 -> EMAT New/2(ERS_V2)
  ERS_V3/1 -> EMAT New/3(ERS_V3)
  ERS_V4/1 -> EMAT New/4(ERS_V4)
  ERS_V5/1 -> EMAT New/5(ERS_V5)
  ERB/1 -> EMAT New/6(ERB), Subtract/2
  DV1/1 -> EMAT New/7(DV1)
  DV2/1 -> EMAT New/8(DV2)
  DV3/1 -> EMAT New/9(DV3)
  DV4/1 -> EMAT New/10(DV4)
  DV5/1 -> EMAT New/11(DV5)
  EMAT New/1(EMAT1) -> EMAT Concatenate/1
  EMAT New/2(EMAT2) -> EMAT Concatenate/2
  EMAT New/3(EMAT3) -> EMAT Concatenate/3
  Subtract/1 -> Matrix Multiply/2
  Add/1 -> Zf/1
  Add1/1 -> Zcl/1
  Add2/1 -> Zch/1
  Add3/1 -> TFth/1
  Add4/1 -> TFtl/1
  EMAT New/4(EMAT4) -> EMAT Concatenate/4
  EMAT New/5(EMAT5) -> EMAT Concatenate/5

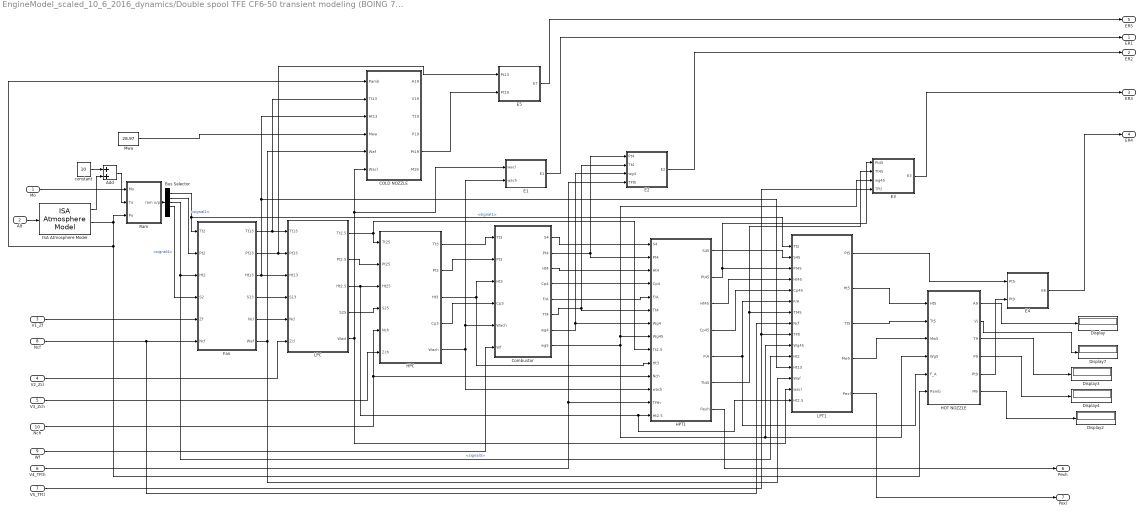
== system EngineModel_scaled_10_6_2016_dynamics/Double spool TFE CF6-50 transient modeling (BOING 747-200)/Error Due to Vs/Error Due To Dv1 ==
  Mo : Inport
  Alt : Inport  Port=2
  V1_Zf : Inport  Port=3
  V2_Zcl : Inport  Port=4
  V3_Zch : Inport  Port=5
  V4_TFth : Inport  Port=6
  V5_TFtl : Inport  Port=7
  Ncf : Inport  Port=8
  Wf : Inport  Port=9
  Nch : Inport  Port=10
  Add : Sum
  Bus Selector : BusSelector  OutputSignals=signal1,signal2,signal3,signal4,signal5
  COLD NOZZLE : Subsystem
  Combustor : Subsystem
  Display{,2..4,7} (5 alike) : Display
  E1 : Subsystem
  E2 : Subsystem
  E3 : Subsystem
  E4 : Subsystem
  E5 : Subsystem
  Fan : Subsystem
  HOT NOZZLE : Subsystem
  HPC : Subsystem
  HPT1 : Subsystem
  ISA Atmosphere Model : aerolibatmos2/ISA Atmosphere Model  custom=on  g=9.81  gamma=1.4  R=287  L=0.0065  h_trop=11000  h_strat=20000  rho0=1.225  P0=101325  T0=288  h0=0
  LPC : Subsystem
  LPT1 : Subsystem
  Mwa : Constant  Value=28.97
  Ram : Subsystem
  constant : Constant  Value=10
  ER1 : Outport
  ER2 : Outport  Port=2
  ER3 : Outport  Port=3
  ER4 : Outport  Port=4
  ER5 : Outport  Port=5
  Pexh : Outport  Port=6
  Pexl : Outport  Port=7
  wires:
  Alt/1 -> ISA Atmosphere Model/1
  Mo/1 -> Ram/1(Mo)
  ISA Atmosphere Model/1 -> Add/2
  Ram/1(ram o/p) -> Bus Selector/1
  ISA Atmosphere Model/3 -> Ram/3(Po), COLD NOZZLE/1(Pamb), HOT NOZZLE/6(Pamb)
  constant/1 -> Add/1
  Add/1 -> Ram/2(To)
  Bus Selector/1 -> LPT1/1(Tt2), Fan/1(Tt2)  "<signal1>"
  Bus Selector/2 -> Fan/2(Pt2)  "<signal2>"
  Fan/1(Tt13) -> LPC/1(Tt13), COLD NOZZLE/2(Tt13)
  Fan/2(Pt13) -> E5/1(Pt13), LPC/2(Pt13)
  LPC/1(Tt2.5) -> HPT1/9(Tt2.5), HPC/1(Tt25)
  LPC/2(Pt2.5) -> HPC/2(Pt25)
  HPC/1(Tt3) -> Combustor/1(Tt3)
  HPC/2(Pt3) -> Combustor/2(Pt3)
  HPC/3(Ht3) -> HPT1/10(Ht3), Combustor/3(Ht3)
  Combustor/2(Pt4) -> E2/1(Pt4), HPT1/2(Pt4)
  Combustor/4(Cp4) -> HPT1/4(Cp4)
  Combustor/5(F/A) -> HPT1/5(F/A)
  Combustor/6(Tt4) -> HPT1/6(Tt4), E2/2(Tt4)
  LPT1/2(Ht5) -> HOT NOZZLE/1(Ht5)
  LPT1/3(Tt5) -> HOT NOZZLE/2(Tt5)
  V1_Zf/1 -> Fan/5(Zf)
  Ncf/1 -> LPT1/8(Ncf), Fan/6(Ncf)
  V2_Zcl/1 -> LPC/6(Zcl)
  V3_Zch/1 -> HPC/6(Zch)
  Nch/1 -> HPC/5(Nch), HPT1/11(Nch)
  Wf/1 -> Combustor/6(Wf)
  V4_TFth/1 -> E2/4(TFth), HPT1/13(TFth)
  Combustor/7(wg4) -> E2/3(wg4), HPT1/7(Wg4)
  LPT1/4(Mw5) -> HOT NOZZLE/3(Mw5)
  Fan/3(Ht13) -> COLD NOZZLE/3(Ht13), LPT1/12(Ht13), LPC/3(Ht13)
  Mwa/1 -> COLD NOZZLE/4(Mwa)
  Fan/6(Waf) -> LPT1/13(Waf), COLD NOZZLE/5(Waf)
  LPC/5(Wacl) -> E1/1(wacl), COLD NOZZLE/6(Wacl), LPT1/14(wacl)
  COLD NOZZLE/5(Pt19) -> E5/2(Pt19)
  LPC/3(Ht2.5) -> HPC/3(Ht25), LPT1/15(Ht2.5), HPT1/14(Ht2.5)
  LPT1/1(Pt5) -> E4/1(Pt5)
  HOT NOZZLE/5(Pt9) -> E4/2(Pt9)
  Combustor/8(wg5) -> E3/3(wg45), HPT1/8(Wg45), LPT1/10(Wg45), HOT NOZZLE/4(Wg5)
  Combustor/3(Ht4) -> HPT1/3(Ht4)
  Combustor/1(S4) -> HPT1/1(S4)
  HOT NOZZLE/1(A9) -> Display/1
  HOT NOZZLE/2(Vj) -> Display7/1
  HOT NOZZLE/3(T9) -> Display3/1
  HOT NOZZLE/4(P9) -> Display4/1
  HOT NOZZLE/6(M9) -> Display2/1
  Bus Selector/3 -> Fan/3(Ht2), LPT1/11(Ht2)  "<signal3>"
  Bus Selector/4 -> Fan/4(S2)  "<signal4>"
  Fan/5(Ncl) -> LPC/5(Ncl)
  Fan/4(S13) -> LPC/4(S13)
  LPC/4(S25) -> HPC/4(S25)
  HPC/5(Wach) -> HPT1/12(wach), Combustor/5(Wach), E1/2(wach)
  HPT1/1(S45) -> LPT1/2(S45)
  HPT1/2(Pt45) -> LPT1/3(Pt45), E3/1(Pt45)
  HPT1/3(Ht45) -> LPT1/4(Ht45)
  HPT1/4(Cp45) -> LPT1/5(Cp45)
  HPT1/6(Tt45) -> LPT1/7(Tt45), E3/2(Tt45)
  HPT1/5(F\A) -> LPT1/6(F/A), HOT NOZZLE/5(F_A)
  V5_TFtl/1 -> LPT1/9(TFtl), E3/4(TFtl)
  E4/1(E6) -> ER4/1
  E3/1(E3) -> ER3/1
  E2/1(E2) -> ER2/1
  E1/1(E1) -> ER1/1
  E5/1(E7) -> ER5/1
  HPC/4(Cp3) -> Combustor/4(Cp3)
  HPT1/7(Pexh) -> Pexh/1
  LPT1/5(Pexl) -> Pexl/1

== system EngineModel_scaled_10_6_2016_dynamics/Double spool TFE CF6-50 transient modeling (BOING 747-200)/Error Due to Vs/Error Due To Dv2 ==
  Mo : Inport
  Alt : Inport  Port=2
  V1_Zf : Inport  Port=3
  V2_Zcl : Inport  Port=4
  V3_Zch : Inport  Port=5
  V4_TFth : Inport  Port=6
  V5_TFtl : Inport  Port=7
  Ncf : Inport  Port=8
  Wf : Inport  Port=9
  Nch : Inport  Port=10
  Add : Sum
  Bus Selector : BusSelector  OutputSignals=signal1,signal2,signal3,signal4,signal5
  COLD NOZZLE : Subsystem
  Combustor : Subsystem
  Display{,2..4,7} (5 alike) : Display
  E1 : Subsystem
  E2 : Subsystem
  E3 : Subsystem
  E4 : Subsystem
  E5 : Subsystem
  Fan : Subsystem
  HOT NOZZLE : Subsystem
  HPC : Subsystem
  HPT : Subsystem
  ISA Atmosphere Model : aerolibatmos2/ISA Atmosphere Model  custom=on  g=9.81  gamma=1.4  R=287  L=0.0065  h_trop=11000  h_strat=20000  rho0=1.225  P0=101325  T0=288  h0=0
  LPC : Subsystem
  LPT : Subsystem
  Mwa : Constant  Value=28.97
  Ram : Subsystem
  constant : Constant  Value=10
  ER1 : Outport
  ER2 : Outport  Port=2
  ER3 : Outport  Port=3
  ER4 : Outport  Port=4
  ER5 : Outport  Port=5
  wires:
  HPC/4(Cp3) -> Combustor/4(Cp3)
  E5/1(E7) -> ER5/1
  E1/1(E1) -> ER1/1
  E2/1(E2) -> ER2/1
  E3/1(E3) -> ER3/1
  E4/1(E6) -> ER4/1
  V5_TFtl/1 -> E3/4(TFtl), LPT/9(TFtl)
  HPT/6(F\A) -> HOT NOZZLE/5(F_A), LPT/6(F/A)
  HPT/7(Tt45) -> E3/2(Tt45), LPT/7(Tt45)
  HPT/5(Cp45) -> LPT/5(Cp45)
  HPT/4(Ht45) -> LPT/4(Ht45)
  HPT/3(Pt45) -> LPT/3(Pt45), E3/1(Pt45)
  HPT/2(S45) -> LPT/2(S45)
  HPC/5(Wach) -> HPT/12(wach), E1/2(wach), Combustor/5(Wach)
  LPC/4(S25) -> HPC/4(S25)
  Fan/4(S13) -> LPC/4(S13)
  Fan/5(Ncl) -> LPC/5(Ncl)
  Bus Selector/4 -> Fan/4(S2)  "<signal4>"
  Bus Selector/3 -> Fan/3(Ht2)  "<signal3>"
  HOT NOZZLE/6(M9) -> Display2/1
  HOT NOZZLE/4(P9) -> Display4/1
  HOT NOZZLE/3(T9) -> Display3/1
  HOT NOZZLE/2(Vj) -> Display7/1
  HOT NOZZLE/1(A9) -> Display/1
  Combustor/1(S4) -> HPT/1(S4)
  Combustor/3(Ht4) -> HPT/3(Ht4)
  Combustor/8(wg5) -> HOT NOZZLE/4(Wg5), HPT/8(Wg45), E3/3(wg45)
  HOT NOZZLE/5(Pt9) -> E4/2(Pt9)
  LPT/2(Pt5) -> E4/1(Pt5)
  LPC/3(Ht2.5) -> HPC/3(Ht25)
  COLD NOZZLE/5(Pt19) -> E5/2(Pt19)
  LPC/5(Wacl) -> E1/1(wacl), COLD NOZZLE/6(Wacl)
  Fan/6(Waf) -> COLD NOZZLE/5(Waf)
  Mwa/1 -> COLD NOZZLE/4(Mwa)
  Fan/3(Ht13) -> LPC/3(Ht13), COLD NOZZLE/3(Ht13)
  LPT/5(Mw5) -> HOT NOZZLE/3(Mw5)
  Combustor/7(wg4) -> HPT/7(Wg4), E2/3(wg4)
  V4_TFth/1 -> HPT/13(TFth), E2/4(TFth)
  Wf/1 -> Combustor/6(Wf)
  Nch/1 -> HPC/5(Nch), HPT/10(Nch)
  V3_Zch/1 -> HPC/6(Zch)
  V2_Zcl/1 -> LPC/6(Zcl)
  Ncf/1 -> Fan/6(Ncf), LPT/8(Ncf)
  V1_Zf/1 -> Fan/5(Zf)
  LPT/4(Tt5) -> HOT NOZZLE/2(Tt5)
  LPT/3(Ht5) -> HOT NOZZLE/1(Ht5)
  Combustor/6(Tt4) -> HPT/6(Tt4), E2/2(Tt4)
  Combustor/5(F/A) -> HPT/5(F/A)
  Combustor/4(Cp4) -> HPT/4(Cp4)
  Combustor/2(Pt4) -> HPT/2(Pt4), E2/1(Pt4)
  HPC/3(Ht3) -> HPT/11(Ht3), Combustor/3(Ht3)
  HPC/2(Pt3) -> Combustor/2(Pt3)
  HPC/1(Tt3) -> Combustor/1(Tt3)
  LPC/2(Pt2.5) -> HPC/2(Pt25)
  LPC/1(Tt2.5) -> HPT/9(Tt2.5), HPC/1(Tt25)
  Fan/2(Pt13) -> LPC/2(Pt13), E5/1(Pt13)
  Fan/1(Tt13) -> COLD NOZZLE/2(Tt13), LPC/1(Tt13)
  Bus Selector/2 -> Fan/2(Pt2)  "<signal2>"
  Bus Selector/1 -> LPT/1(Tt2), Fan/1(Tt2)  "<signal1>"
  Add/1 -> Ram/2(To)
  constant/1 -> Add/1
  ISA Atmosphere Model/3 -> HOT NOZZLE/6(Pamb), COLD NOZZLE/1(Pamb), Ram/3(Po)
  Ram/1(ram o/p) -> Bus Selector/1
  ISA Atmosphere Model/1 -> Add/2
  Mo/1 -> Ram/1(Mo)
  Alt/1 -> ISA Atmosphere Model/1

== system EngineModel_scaled_10_6_2016_dynamics/Double spool TFE CF6-50 transient modeling (BOING 747-200)/Error Due to Vs/Error Due To Dv3 ==
  Mo : Inport
  Alt : Inport  Port=2
  V1_Zf : Inport  Port=3
  V2_Zcl : Inport  Port=4
  V3_Zch : Inport  Port=5
  V4_TFth : Inport  Port=6
  V5_TFtl : Inport  Port=7
  Ncf : Inport  Port=8
  Wf : Inport  Port=9
  Nch : Inport  Port=10
  Add : Sum
  Bus Selector : BusSelector  OutputSignals=signal1,signal2,signal3,signal4,signal5
  COLD NOZZLE : Subsystem
  Combustor : Subsystem
  Display{,2..4,7} (5 alike) : Display
  E1 : Subsystem
  E2 : Subsystem
  E3 : Subsystem
  E4 : Subsystem
  E5 : Subsystem
  Fan : Subsystem
  HOT NOZZLE : Subsystem
  HPC : Subsystem
  HPT : Subsystem
  ISA Atmosphere Model : aerolibatmos2/ISA Atmosphere Model  custom=on  g=9.81  gamma=1.4  R=287  L=0.0065  h_trop=11000  h_strat=20000  rho0=1.225  P0=101325  T0=288  h0=0
  LPC : Subsystem
  LPT : Subsystem
  Mwa : Constant  Value=28.97
  Ram : Subsystem
  constant : Constant  Value=10
  ER1 : Outport
  ER2 : Outport  Port=2
  ER3 : Outport  Port=3
  ER4 : Outport  Port=4
  ER5 : Outport  Port=5
  wires:
  Alt/1 -> ISA Atmosphere Model/1
  Mo/1 -> Ram/1(Mo)
  ISA Atmosphere Model/1 -> Add/2
  Ram/1(ram o/p) -> Bus Selector/1
  ISA Atmosphere Model/3 -> Ram/3(Po), COLD NOZZLE/1(Pamb), HOT NOZZLE/6(Pamb)
  constant/1 -> Add/1
  Add/1 -> Ram/2(To)
  Bus Selector/1 -> Fan/1(Tt2), LPT/1(Tt2)  "<signal1>"
  Bus Selector/2 -> Fan/2(Pt2)  "<signal2>"
  Fan/1(Tt13) -> LPC/1(Tt13), COLD NOZZLE/2(Tt13)
  Fan/2(Pt13) -> E5/1(Pt13), LPC/2(Pt13)
  LPC/1(Tt2.5) -> HPC/1(Tt25), HPT/9(Tt2.5)
  LPC/2(Pt2.5) -> HPC/2(Pt25)
  HPC/1(Tt3) -> Combustor/1(Tt3)
  HPC/2(Pt3) -> Combustor/2(Pt3)
  HPC/3(Ht3) -> Combustor/3(Ht3), HPT/11(Ht3)
  Combustor/2(Pt4) -> E2/1(Pt4), HPT/2(Pt4)
  Combustor/4(Cp4) -> HPT/4(Cp4)
  Combustor/5(F/A) -> HPT/5(F/A)
  Combustor/6(Tt4) -> E2/2(Tt4), HPT/6(Tt4)
  LPT/3(Ht5) -> HOT NOZZLE/1(Ht5)
  LPT/4(Tt5) -> HOT NOZZLE/2(Tt5)
  V1_Zf/1 -> Fan/5(Zf)
  Ncf/1 -> LPT/8(Ncf), Fan/6(Ncf)
  V2_Zcl/1 -> LPC/6(Zcl)
  V3_Zch/1 -> HPC/6(Zch)
  Nch/1 -> HPT/10(Nch), HPC/5(Nch)
  Wf/1 -> Combustor/6(Wf)
  V4_TFth/1 -> E2/4(TFth), HPT/13(TFth)
  Combustor/7(wg4) -> E2/3(wg4), HPT/7(Wg4)
  LPT/5(Mw5) -> HOT NOZZLE/3(Mw5)
  Fan/3(Ht13) -> COLD NOZZLE/3(Ht13), LPC/3(Ht13)
  Mwa/1 -> COLD NOZZLE/4(Mwa)
  Fan/6(Waf) -> COLD NOZZLE/5(Waf)
  LPC/5(Wacl) -> COLD NOZZLE/6(Wacl), E1/1(wacl)
  COLD NOZZLE/5(Pt19) -> E5/2(Pt19)
  LPC/3(Ht2.5) -> HPC/3(Ht25)
  LPT/2(Pt5) -> E4/1(Pt5)
  HOT NOZZLE/5(Pt9) -> E4/2(Pt9)
  Combustor/8(wg5) -> E3/3(wg45), HPT/8(Wg45), HOT NOZZLE/4(Wg5)
  Combustor/3(Ht4) -> HPT/3(Ht4)
  Combustor/1(S4) -> HPT/1(S4)
  HOT NOZZLE/1(A9) -> Display/1
  HOT NOZZLE/2(Vj) -> Display7/1
  HOT NOZZLE/3(T9) -> Display3/1
  HOT NOZZLE/4(P9) -> Display4/1
  HOT NOZZLE/6(M9) -> Display2/1
  Bus Selector/3 -> Fan/3(Ht2)  "<signal3>"
  Bus Selector/4 -> Fan/4(S2)  "<signal4>"
  Fan/5(Ncl) -> LPC/5(Ncl)
  Fan/4(S13) -> LPC/4(S13)
  LPC/4(S25) -> HPC/4(S25)
  HPC/5(Wach) -> Combustor/5(Wach), E1/2(wach), HPT/12(wach)
  HPT/2(S45) -> LPT/2(S45)
  HPT/3(Pt45) -> E3/1(Pt45), LPT/3(Pt45)
  HPT/4(Ht45) -> LPT/4(Ht45)
  HPT/5(Cp45) -> LPT/5(Cp45)
  HPT/7(Tt45) -> LPT/7(Tt45), E3/2(Tt45)
  HPT/6(F\A) -> LPT/6(F/A), HOT NOZZLE/5(F_A)
  V5_TFtl/1 -> LPT/9(TFtl), E3/4(TFtl)
  E4/1(E6) -> ER4/1
  E3/1(E3) -> ER3/1
  E2/1(E2) -> ER2/1
  E1/1(E1) -> ER1/1
  E5/1(E7) -> ER5/1
  HPC/4(Cp3) -> Combustor/4(Cp3)

== system EngineModel_scaled_10_6_2016_dynamics/Double spool TFE CF6-50 transient modeling (BOING 747-200)/Error Due to Vs/Error Due To Dv4 ==
  Mo : Inport
  Alt : Inport  Port=2
  V1_Zf : Inport  Port=3
  V2_Zcl : Inport  Port=4
  V3_Zch : Inport  Port=5
  V4_TFth : Inport  Port=6
  V5_TFtl : Inport  Port=7
  Ncf : Inport  Port=8
  Wf : Inport  Port=9
  Nch : Inport  Port=10
  Add : Sum
  Bus Selector : BusSelector  OutputSignals=signal1,signal2,signal3,signal4,signal5
  COLD NOZZLE : Subsystem
  Combustor : Subsystem
  Display{,2..4,7} (5 alike) : Display
  E1 : Subsystem
  E2 : Subsystem
  E3 : Subsystem
  E4 : Subsystem
  E5 : Subsystem
  Fan : Subsystem
  HOT NOZZLE : Subsystem
  HPC : Subsystem
  HPT : Subsystem
  ISA Atmosphere Model : aerolibatmos2/ISA Atmosphere Model  custom=on  g=9.81  gamma=1.4  R=287  L=0.0065  h_trop=11000  h_strat=20000  rho0=1.225  P0=101325  T0=288  h0=0
  LPC : Subsystem
  LPT : Subsystem
  Mwa : Constant  Value=28.97
  Ram : Subsystem
  constant : Constant  Value=10
  ER1 : Outport
  ER2 : Outport  Port=2
  ER3 : Outport  Port=3
  ER4 : Outport  Port=4
  ER5 : Outport  Port=5
  wires:
  HPC/4(Cp3) -> Combustor/4(Cp3)
  E5/1(E7) -> ER5/1
  E1/1(E1) -> ER1/1
  E2/1(E2) -> ER2/1
  E3/1(E3) -> ER3/1
  E4/1(E6) -> ER4/1
  V5_TFtl/1 -> E3/4(TFtl), LPT/9(TFtl)
  HPT/6(F\A) -> HOT NOZZLE/5(F_A), LPT/6(F/A)
  HPT/7(Tt45) -> E3/2(Tt45), LPT/7(Tt45)
  HPT/5(Cp45) -> LPT/5(Cp45)
  HPT/4(Ht45) -> LPT/4(Ht45)
  HPT/3(Pt45) -> LPT/3(Pt45), E3/1(Pt45)
  HPT/2(S45) -> LPT/2(S45)
  HPC/5(Wach) -> HPT/12(wach), E1/2(wach), Combustor/5(Wach)
  LPC/4(S25) -> HPC/4(S25)
  Fan/4(S13) -> LPC/4(S13)
  Fan/5(Ncl) -> LPC/5(Ncl)
  Bus Selector/4 -> Fan/4(S2)  "<signal4>"
  Bus Selector/3 -> Fan/3(Ht2)  "<signal3>"
  HOT NOZZLE/6(M9) -> Display2/1
  HOT NOZZLE/4(P9) -> Display4/1
  HOT NOZZLE/3(T9) -> Display3/1
  HOT NOZZLE/2(Vj) -> Display7/1
  HOT NOZZLE/1(A9) -> Display/1
  Combustor/1(S4) -> HPT/1(S4)
  Combustor/3(Ht4) -> HPT/3(Ht4)
  Combustor/8(wg5) -> HOT NOZZLE/4(Wg5), HPT/8(Wg45), E3/3(wg45)
  HOT NOZZLE/5(Pt9) -> E4/2(Pt9)
  LPT/2(Pt5) -> E4/1(Pt5)
  LPC/3(Ht2.5) -> HPC/3(Ht25)
  COLD NOZZLE/5(Pt19) -> E5/2(Pt19)
  LPC/5(Wacl) -> E1/1(wacl), COLD NOZZLE/6(Wacl)
  Fan/6(Waf) -> COLD NOZZLE/5(Waf)
  Mwa/1 -> COLD NOZZLE/4(Mwa)
  Fan/3(Ht13) -> LPC/3(Ht13), COLD NOZZLE/3(Ht13)
  LPT/5(Mw5) -> HOT NOZZLE/3(Mw5)
  Combustor/7(wg4) -> HPT/7(Wg4), E2/3(wg4)
  V4_TFth/1 -> HPT/13(TFth), E2/4(TFth)
  Wf/1 -> Combustor/6(Wf)
  Nch/1 -> HPC/5(Nch), HPT/10(Nch)
  V3_Zch/1 -> HPC/6(Zch)
  V2_Zcl/1 -> LPC/6(Zcl)
  Ncf/1 -> Fan/6(Ncf), LPT/8(Ncf)
  V1_Zf/1 -> Fan/5(Zf)
  LPT/4(Tt5) -> HOT NOZZLE/2(Tt5)
  LPT/3(Ht5) -> HOT NOZZLE/1(Ht5)
  Combustor/6(Tt4) -> HPT/6(Tt4), E2/2(Tt4)
  Combustor/5(F/A) -> HPT/5(F/A)
  Combustor/4(Cp4) -> HPT/4(Cp4)
  Combustor/2(Pt4) -> HPT/2(Pt4), E2/1(Pt4)
  HPC/3(Ht3) -> HPT/11(Ht3), Combustor/3(Ht3)
  HPC/2(Pt3) -> Combustor/2(Pt3)
  HPC/1(Tt3) -> Combustor/1(Tt3)
  LPC/2(Pt2.5) -> HPC/2(Pt25)
  LPC/1(Tt2.5) -> HPT/9(Tt2.5), HPC/1(Tt25)
  Fan/2(Pt13) -> LPC/2(Pt13), E5/1(Pt13)
  Fan/1(Tt13) -> COLD NOZZLE/2(Tt13), LPC/1(Tt13)
  Bus Selector/2 -> Fan/2(Pt2)  "<signal2>"
  Bus Selector/1 -> LPT/1(Tt2), Fan/1(Tt2)  "<signal1>"
  Add/1 -> Ram/2(To)
  constant/1 -> Add/1
  ISA Atmosphere Model/3 -> HOT NOZZLE/6(Pamb), COLD NOZZLE/1(Pamb), Ram/3(Po)
  Ram/1(ram o/p) -> Bus Selector/1
  ISA Atmosphere Model/1 -> Add/2
  Mo/1 -> Ram/1(Mo)
  Alt/1 -> ISA Atmosphere Model/1

== system EngineModel_scaled_10_6_2016_dynamics/Double spool TFE CF6-50 transient modeling (BOING 747-200)/Error Due to Vs/Error Due To Dv5 ==
  Mo : Inport
  Alt : Inport  Port=2
  V1_Zf : Inport  Port=3
  V2_Zcl : Inport  Port=4
  V3_Zch : Inport  Port=5
  V4_TFth : Inport  Port=6
  V5_TFtl : Inport  Port=7
  Ncf : Inport  Port=8
  Wf : Inport  Port=9
  Nch : Inport  Port=10
  Add : Sum
  Bus Selector : BusSelector  OutputSignals=signal1,signal2,signal3,signal4,signal5
  COLD NOZZLE : Subsystem
  Combustor : Subsystem
  Display{,2..4,7} (5 alike) : Display
  E1 : Subsystem
  E2 : Subsystem
  E3 : Subsystem
  E4 : Subsystem
  E5 : Subsystem
  Fan : Subsystem
  HOT NOZZLE : Subsystem
  HPC : Subsystem
  HPT : Subsystem
  ISA Atmosphere Model : aerolibatmos2/ISA Atmosphere Model  custom=on  g=9.81  gamma=1.4  R=287  L=0.0065  h_trop=11000  h_strat=20000  rho0=1.225  P0=101325  T0=288  h0=0
  LPC : Subsystem
  LPT : Subsystem
  Mwa : Constant  Value=28.97
  Ram : Subsystem
  constant : Constant  Value=10
  ER1 : Outport
  ER2 : Outport  Port=2
  ER3 : Outport  Port=3
  ER4 : Outport  Port=4
  ER5 : Outport  Port=5
  wires:
  Alt/1 -> ISA Atmosphere Model/1
  Mo/1 -> Ram/1(Mo)
  ISA Atmosphere Model/1 -> Add/2
  Ram/1(ram o/p) -> Bus Selector/1
  ISA Atmosphere Model/3 -> Ram/3(Po), COLD NOZZLE/1(Pamb), HOT NOZZLE/6(Pamb)
  constant/1 -> Add/1
  Add/1 -> Ram/2(To)
  Bus Selector/1 -> Fan/1(Tt2), LPT/1(Tt2)  "<signal1>"
  Bus Selector/2 -> Fan/2(Pt2)  "<signal2>"
  Fan/1(Tt13) -> LPC/1(Tt13), COLD NOZZLE/2(Tt13)
  Fan/2(Pt13) -> E5/1(Pt13), LPC/2(Pt13)
  LPC/1(Tt2.5) -> HPC/1(Tt25), HPT/9(Tt2.5)
  LPC/2(Pt2.5) -> HPC/2(Pt25)
  HPC/1(Tt3) -> Combustor/1(Tt3)
  HPC/2(Pt3) -> Combustor/2(Pt3)
  HPC/3(Ht3) -> Combustor/3(Ht3), HPT/11(Ht3)
  Combustor/2(Pt4) -> E2/1(Pt4), HPT/2(Pt4)
  Combustor/4(Cp4) -> HPT/4(Cp4)
  Combustor/5(F/A) -> HPT/5(F/A)
  Combustor/6(Tt4) -> E2/2(Tt4), HPT/6(Tt4)
  LPT/3(Ht5) -> HOT NOZZLE/1(Ht5)
  LPT/4(Tt5) -> HOT NOZZLE/2(Tt5)
  V1_Zf/1 -> Fan/5(Zf)
  Ncf/1 -> LPT/8(Ncf), Fan/6(Ncf)
  V2_Zcl/1 -> LPC/6(Zcl)
  V3_Zch/1 -> HPC/6(Zch)
  Nch/1 -> HPT/10(Nch), HPC/5(Nch)
  Wf/1 -> Combustor/6(Wf)
  V4_TFth/1 -> E2/4(TFth), HPT/13(TFth)
  Combustor/7(wg4) -> E2/3(wg4), HPT/7(Wg4)
  LPT/5(Mw5) -> HOT NOZZLE/3(Mw5)
  Fan/3(Ht13) -> COLD NOZZLE/3(Ht13), LPC/3(Ht13)
  Mwa/1 -> COLD NOZZLE/4(Mwa)
  Fan/6(Waf) -> COLD NOZZLE/5(Waf)
  LPC/5(Wacl) -> COLD NOZZLE/6(Wacl), E1/1(wacl)
  COLD NOZZLE/5(Pt19) -> E5/2(Pt19)
  LPC/3(Ht2.5) -> HPC/3(Ht25)
  LPT/2(Pt5) -> E4/1(Pt5)
  HOT NOZZLE/5(Pt9) -> E4/2(Pt9)
  Combustor/8(wg5) -> E3/3(wg45), HPT/8(Wg45), HOT NOZZLE/4(Wg5)
  Combustor/3(Ht4) -> HPT/3(Ht4)
  Combustor/1(S4) -> HPT/1(S4)
  HOT NOZZLE/1(A9) -> Display/1
  HOT NOZZLE/2(Vj) -> Display7/1
  HOT NOZZLE/3(T9) -> Display3/1
  HOT NOZZLE/4(P9) -> Display4/1
  HOT NOZZLE/6(M9) -> Display2/1
  Bus Selector/3 -> Fan/3(Ht2)  "<signal3>"
  Bus Selector/4 -> Fan/4(S2)  "<signal4>"
  Fan/5(Ncl) -> LPC/5(Ncl)
  Fan/4(S13) -> LPC/4(S13)
  LPC/4(S25) -> HPC/4(S25)
  HPC/5(Wach) -> Combustor/5(Wach), E1/2(wach), HPT/12(wach)
  HPT/2(S45) -> LPT/2(S45)
  HPT/3(Pt45) -> E3/1(Pt45), LPT/3(Pt45)
  HPT/4(Ht45) -> LPT/4(Ht45)
  HPT/5(Cp45) -> LPT/5(Cp45)
  HPT/7(Tt45) -> LPT/7(Tt45), E3/2(Tt45)
  HPT/6(F\A) -> LPT/6(F/A), HOT NOZZLE/5(F_A)
  V5_TFtl/1 -> LPT/9(TFtl), E3/4(TFtl)
  E4/1(E6) -> ER4/1
  E3/1(E3) -> ER3/1
  E2/1(E2) -> ER2/1
  E1/1(E1) -> ER1/1
  E5/1(E7) -> ER5/1
  HPC/4(Cp3) -> Combustor/4(Cp3)

== system EngineModel_scaled_10_6_2016_dynamics/Double spool TFE CF6-50 transient modeling (BOING 747-200)/Off- Design Module/COLD NOZZLE ==
  Po : Inport
  Tt13 : Inport  Port=2
  Ht13 : Inport  Port=3
  Mwa : Inport  Port=4
  Waf : Inport  Port=5
  Wacl : Inport  Port=6
  Demux : Demux  Outputs=6
  Display : Display
  Display1 : Display
  Interpreted MATLAB Function : MATLABFcn  MATLABFcn=coldnozzle(u(1),u(2),u(3),u(4),u(5),u(6))  OutputDimensions=6
  Mux : Mux  Inputs=6
      settings: DisplayOption=signals
  A19 : Outport
  V19 : Outport  Port=2
  T19 : Outport  Port=3
  P19 : Outport  Port=4
  Pt19 : Outport  Port=5
  M19 : Outport  Port=6
  wires:
  Mux/1 -> Interpreted MATLAB Function/1
  Interpreted MATLAB Function/1 -> Demux/1
  Ht13/1 -> Mux/3
  Mwa/1 -> Mux/4
  Waf/1 -> Mux/5
  Wacl/1 -> Mux/6
  Demux/1 -> A19/1
  Demux/2 -> Display/1, V19/1
  Demux/3 -> Display1/1, T19/1
  Demux/4 -> P19/1
  Demux/5 -> Pt19/1
  Demux/6 -> M19/1
  Tt13/1 -> Mux/2
  Po/1 -> Mux/1

== system EngineModel_scaled_10_6_2016_dynamics/Double spool TFE CF6-50 transient modeling (BOING 747-200)/Off- Design Module/Combustor ==
  Tt3 : Inport
  Pt3 : Inport  Port=2
  Ht3 : Inport  Port=3
  Cp3 : Inport  Port=4
  Wach : Inport  Port=5
  Wf : Inport  Port=6
  (1-percent bleed airpcwb2) : Constant  Value=0.9
  Add1 : Sum
  Add2 : Sum
  Display{1..2,4..7} (6 alike) : Display
  Product : Product
  Thermo_combustor : Subsystem  TreatAsAtomicUnit=on
  combustor o/p enthalpy : Subsystem  TreatAsAtomicUnit=on
  combustor o/p pressure : Subsystem
  S4 : Outport
  Pt4 : Outport  Port=2
  Ht4 : Outport  Port=3
  Cp4 : Outport  Port=4
  F/A : Outport  Port=5
  Tt4 : Outport  Port=6
  wg4 : Outport  Port=7
  wg5 : Outport  Port=8
  wires:
  Pt3/1 -> combustor o/p pressure/1(Pt3)
  Tt3/1 -> combustor o/p pressure/2(Tt3)
  Wf/1 -> Add1/2, Add2/2, combustor o/p enthalpy/1("wf ")
  Ht3/1 -> combustor o/p enthalpy/3(Ht3)
  combustor o/p pressure/1(Pt4) -> Display1/1, Pt4/1, Thermo_combustor/1(Pt4)
  combustor o/p enthalpy/2(F_A) -> F/A/1, Thermo_combustor/4(F/A)
  Thermo_combustor/2(S4) -> Display7/1, S4/1
  Thermo_combustor/3(Cp4) -> Cp4/1
  Thermo_combustor/1(Tt4) -> Tt4/1, Display4/1
  Add1/1 -> Display2/1, wg5/1
  Wach/1 -> Product/2, combustor o/p pressure/3(wach), combustor o/p enthalpy/2(wach), Add1/1
  combustor o/p enthalpy/1(Ht4) -> Ht4/1, Display5/1, Thermo_combustor/3("Ht4 ")
  Product/1 -> Add2/1
  (1-percent bleed airpcwb2)/1 -> Product/1
  Add2/1 -> Display6/1, combustor o/p enthalpy/4(wg4), wg4/1
  Cp3/1 -> Thermo_combustor/2(Cp3)

== system EngineModel_scaled_10_6_2016_dynamics/Double spool TFE CF6-50 transient modeling (BOING 747-200)/Off- Design Module/E1 ==
  wacl : Inport
  wach : Inport  Port=2
  Abs : Abs
  Data Type Conversion : DataTypeConversion  OutDataTypeStr=boolean
  Display : Display
  Divide1 : Product  Inputs=*/
  Sum : Sum  Inputs=-+  SaturateOnIntegerOverflow=on
  condition : Subsystem
  E1 : Outport
  cond1 : Outport  Port=2  OutDataTypeStr=boolean
  wires:
  wacl/1 -> Sum/1
  wach/1 -> Divide1/2, Sum/2
  Sum/1 -> Divide1/1
  Abs/1 -> condition/1(In1)
  Data Type Conversion/1 -> cond1/1
  condition/1(Out1) -> Data Type Conversion/1
  Divide1/1 -> Display/1, Abs/1, E1/1

== system EngineModel_scaled_10_6_2016_dynamics/Double spool TFE CF6-50 transient modeling (BOING 747-200)/Off- Design Module/E2 ==
  Pt4 : Inport
  Tt4 : Inport  Port=2
  wg4 : Inport  Port=3
  TFth : Inport  Port=4
  Abs : Abs
  Constant : Constant  Value=100000
  Data Type Conversion : DataTypeConversion  OutDataTypeStr=boolean
  Display{,1..4} (5 alike) : Display
  Divide1 : Product  Inputs=/*
  Divide2 : Product  Inputs=/*
  Divide3 : Product  Inputs=/*
  Product5 : Product  Inputs=**  SaturateOnIntegerOverflow=on  OutDataTypeStr=Inherit: Same as first input
  Sqrt1 : Sqrt  SaturateOnIntegerOverflow=on
  Sum : Sum  Inputs=+-  SaturateOnIntegerOverflow=on
  condition : Subsystem
  E2 : Outport
  cond2 : Outport  Port=2  OutDataTypeStr=boolean
  wires:
  Sum/1 -> Divide1/2
  TFth/1 -> Display1/1, Sum/2
  Divide2/1 -> Sum/1, Display2/1, Divide1/1
  Tt4/1 -> Sqrt1/1
  wg4/1 -> Display3/1, Product5/2
  Sqrt1/1 -> Product5/1
  Product5/1 -> Divide2/2
  Pt4/1 -> Divide3/2
  Constant/1 -> Divide3/1
  Divide3/1 -> Divide2/1, Display4/1
  Abs/1 -> condition/1(In1)
  Data Type Conversion/1 -> cond2/1
  condition/1(Out1) -> Data Type Conversion/1
  Divide1/1 -> Abs/1, E2/1, Display/1

== system EngineModel_scaled_10_6_2016_dynamics/Double spool TFE CF6-50 transient modeling (BOING 747-200)/Off- Design Module/E3 ==
  Pt45 : Inport
  Tt45 : Inport  Port=2
  wg45 : Inport  Port=3
  TFtl : Inport  Port=4
  Abs : Abs
  Constant : Constant  Value=100000
  Data Type Conversion : DataTypeConversion  OutDataTypeStr=boolean
  Display : Display
  Display1 : Display
  Divide1 : Product  Inputs=/*
  Divide2 : Product  Inputs=/*
  Divide3 : Product  Inputs=/*
  Product5 : Product  Inputs=**  SaturateOnIntegerOverflow=on  OutDataTypeStr=Inherit: Same as first input
  Sqrt1 : Sqrt  SaturateOnIntegerOverflow=on
  Sum : Sum  Inputs=+-  SaturateOnIntegerOverflow=on
  condition : Subsystem
  E4 : Outport
  cond4 : Outport  Port=2  OutDataTypeStr=boolean
  wires:
  Product5/1 -> Divide2/2
  Sqrt1/1 -> Product5/1
  wg45/1 -> Product5/2
  Tt45/1 -> Sqrt1/1
  Divide2/1 -> Sum/1, Divide1/1, Display1/1
  TFtl/1 -> Sum/2
  Sum/1 -> Divide1/2
  Pt45/1 -> Divide3/2
  Constant/1 -> Divide3/1
  Divide3/1 -> Divide2/1
  Abs/1 -> condition/1(In1)
  Data Type Conversion/1 -> cond4/1
  condition/1(Out1) -> Data Type Conversion/1
  Divide1/1 -> Abs/1, E4/1, Display/1
